simulink model "cstrseries (1)"  (R2024a)
settings: Solver=VariableStepAuto  StartTime=0.0  StopTime=10.0  RelTol=1e-3

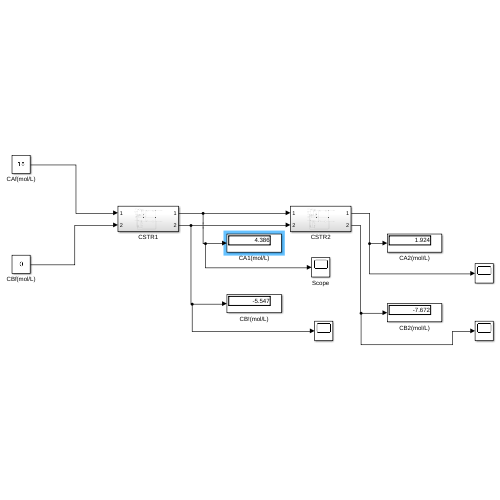
[thumbnail: Simulink's stored preview of the top-level diagram]
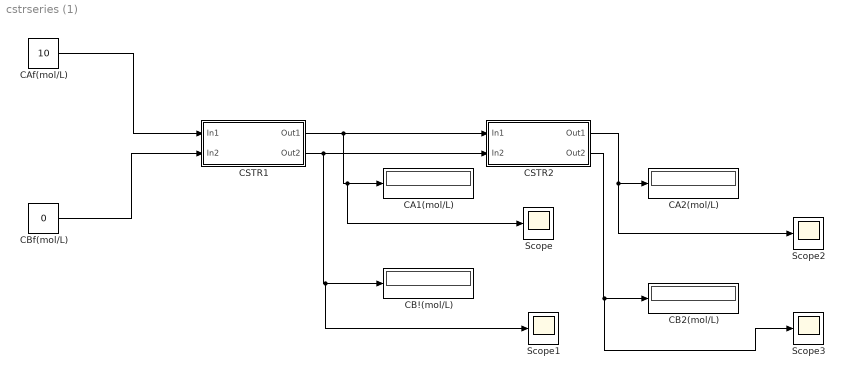
== system cstrseries (1) ==
  CA1(mol/L) : Display
  CA2(mol/L) : Display
  CAf(mol/L) : Constant  Value=10
  CB!(mol/L) : Display
  CB2(mol/L) : Display
  CBf(mol/L) : Constant  Value=0
  CSTR1 : Subsystem
  CSTR2 : Subsystem
  Scope{,1..3} (4 alike) : Scope
  wires:
  CAf(mol/L)/1 -> CSTR1/1(In1)
  CBf(mol/L)/1 -> CSTR1/2(In2)
  CSTR1/1(Out1) -> CSTR2/1(In1), CA1(mol/L)/1, Scope/1
  CSTR1/2(Out2) -> CSTR2/2(In2), Scope1/1, CB!(mol/L)/1
  CSTR2/1(Out1) -> Scope2/1, CA2(mol/L)/1
  CSTR2/2(Out2) -> Scope3/1, CB2(mol/L)/1

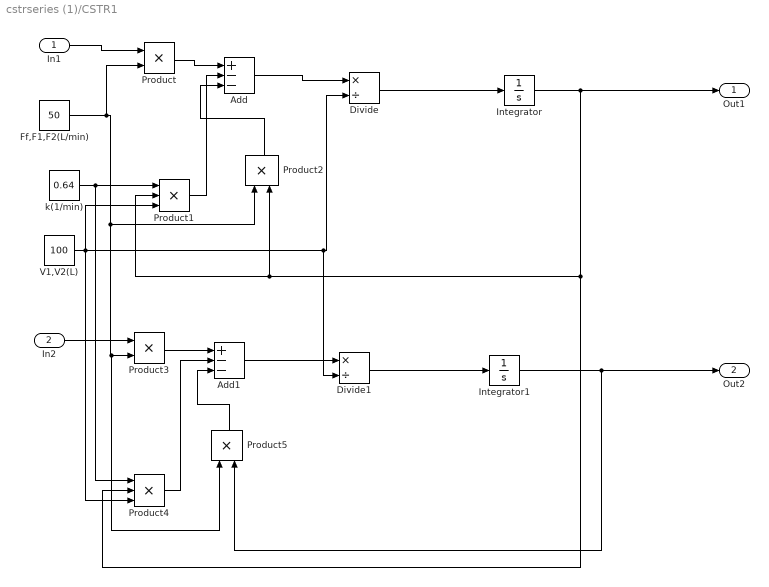
== system cstrseries (1)/CSTR1 ==
  In1 : Inport
  In2 : Inport  Port=2
  Add : Sum  Inputs=+--
  Add1 : Sum  Inputs=+--
  Divide : Product  Inputs=*/
  Divide1 : Product  Inputs=*/
  Ff,F1,F2(L/min) : Constant  Value=50
  Integrator : Integrator  InitialCondition=10
  Integrator1 : Integrator  InitialCondition=10
  Product{,2..3,5} (4 alike) : Product
  Product1 : Product  Inputs=3
  Product4 : Product  Inputs=3
  V1,V2(L) : Constant  Value=100
  k(1/min) : Constant  Value=0.64
  Out1 : Outport
  Out2 : Outport  Port=2
  wires:
  In1/1 -> Product/1
  Ff,F1,F2(L/min)/1 -> Product5/1, Product3/2, Product2/1, Product/2
  Product/1 -> Add/1
  Add/1 -> Divide/1
  V1,V2(L)/1 -> Product4/3, Product1/3, Divide1/2, Divide/2
  Divide/1 -> Integrator/1
  Integrator/1 -> Out1/1, Product4/2, Product2/2, Product1/2
  k(1/min)/1 -> Product4/1, Product1/1
  Product1/1 -> Add/2
  Product2/1 -> Add/3
  In2/1 -> Product3/1
  Product3/1 -> Add1/1
  Add1/1 -> Divide1/1
  Divide1/1 -> Integrator1/1
  Integrator1/1 -> Out2/1, Product5/2
  Product5/1 -> Add1/3
  Product4/1 -> Add1/2

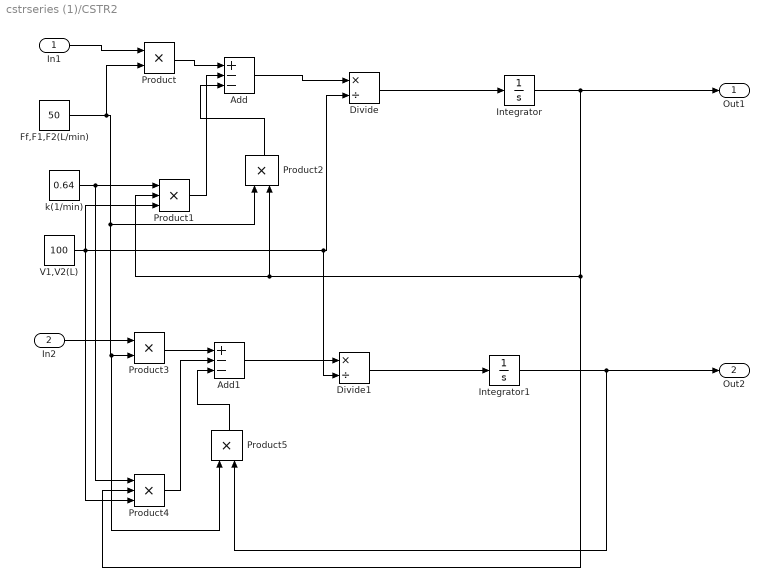
== system cstrseries (1)/CSTR2 ==
  In1 : Inport
  In2 : Inport  Port=2
  Add : Sum  Inputs=+--
  Add1 : Sum  Inputs=+--
  Divide : Product  Inputs=*/
  Divide1 : Product  Inputs=*/
  Ff,F1,F2(L/min) : Constant  Value=50
  Integrator : Integrator  InitialCondition=10
  Integrator1 : Integrator  InitialCondition=10
  Product{,2..3,5} (4 alike) : Product
  Product1 : Product  Inputs=3
  Product4 : Product  Inputs=3
  V1,V2(L) : Constant  Value=100
  k(1/min) : Constant  Value=0.64
  Out1 : Outport
  Out2 : Outport  Port=2
  wires:
  In1/1 -> Product/1
  Ff,F1,F2(L/min)/1 -> Product5/1, Product3/2, Product2/1, Product/2
  Product/1 -> Add/1
  Add/1 -> Divide/1
  V1,V2(L)/1 -> Product4/3, Product1/3, Divide1/2, Divide/2
  Divide/1 -> Integrator/1
  Integrator/1 -> Out1/1, Product4/2, Product2/2, Product1/2
  k(1/min)/1 -> Product4/1, Product1/1
  Product1/1 -> Add/2
  Product2/1 -> Add/3
  In2/1 -> Product3/1
  Product3/1 -> Add1/1
  Add1/1 -> Divide1/1
  Divide1/1 -> Integrator1/1
  Integrator1/1 -> Out2/1, Product5/2
  Product5/1 -> Add1/3
  Product4/1 -> Add1/2
